simulink subsystem "LowLevelControllerSUB2022"  (R2022b)
settings: Solver=VariableStepAuto  StartTime=0.0  StopTime=10.0  RelTol=1e-3
undefined symbols (not defined in the file): km
settings Model: Creator=romav  LastModifiedBy=romav
settings OptimizationCC: ReuseModelBlockBuffer=on

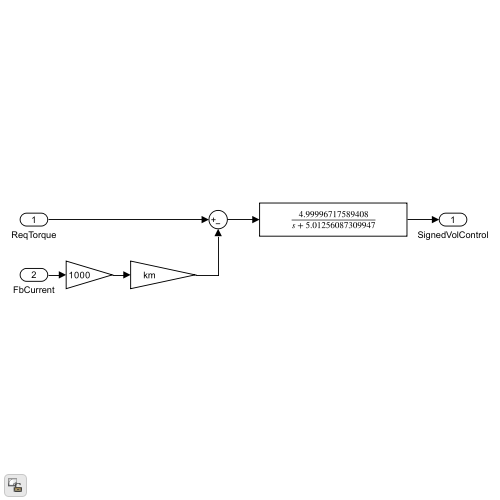
[thumbnail: Simulink's stored preview of the top-level diagram]
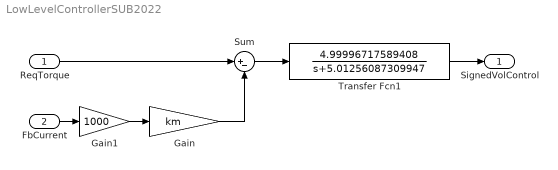
== system LowLevelControllerSUB2022 ==
  ReqTorque : Inport
  FbCurrent : Inport  Port=2
  Gain : Gain  Gain=km
  Gain1 : Gain  Gain=1000
  Sum : Sum  Inputs=|+-
  Transfer Fcn1 : TransferFcn  Numerator=[0 4.99996717589408]  Denominator=[1 5.01256087309947]
  SignedVolControl : Outport
  wires:
  Gain/1 -> Sum/2
  Transfer Fcn1/1 -> SignedVolControl/1
  Sum/1 -> Transfer Fcn1/1
  ReqTorque/1 -> Sum/1
  FbCurrent/1 -> Gain1/1
  Gain1/1 -> Gain/1
